simulink model "DcMotorSimulink"  (R2025a)
settings: Solver=FixedStepAuto  StartTime=0.0  StopTime=10  FixedStep=1e-4  RelTol=1e-3
undefined symbols (not defined in the file): bm, Jm, Kphi, La, Ra
settings Model: DataDictionary=DcMotor.sldd  Creator=tecnicomcbti  LastModifiedBy=tecnicomcbti
settings SolverCC: ConcurrentTasks=on  PositivePriorityOrder=on
settings OptimizationCC: BlockReduction=off  OptimizeBlockIOStorage=off
settings DebuggingCC: AlgebraicLoopMsg=none  TasksWithSamePriorityMsg=none
settings HardwareCC: ProdBitPerLong=64.0  ProdLongLongMode=on  ProdHWDeviceType=Intel->x86-64 (Linux 64)
settings RTWCC: SystemTargetFile=speedgoat.tlc  TemplateMakefile=slrealtime_default_tmf  Toolchain=Simulink Real-Time Toolchain  BuildConfiguration=Faster Runs  CodeExecutionProfiling=on  TargetLang=C++  Description=Speedgoat Real-Time Target Machine
settings SimulinkRealTimeTargetCC: SLRTFileLogMaxRuns=1.0  ExtModeMaxTrigDuration=10.0  ExtModeStaticAllocSize=1000000.0  ExtModeTransport=0.0  MultiwordLength=2048.0  DynamicStringBufferSize=256.0  PreserveMATLABNamespacesInGeneratedCode=on  SubcomponentCodeInterfacePackaging=Reusable function  InstructionSetFMA=off  LogToMDFFile=off

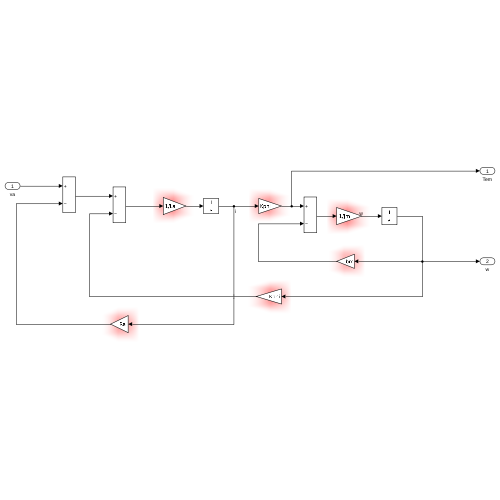
[thumbnail: Simulink's stored preview of the top-level diagram]
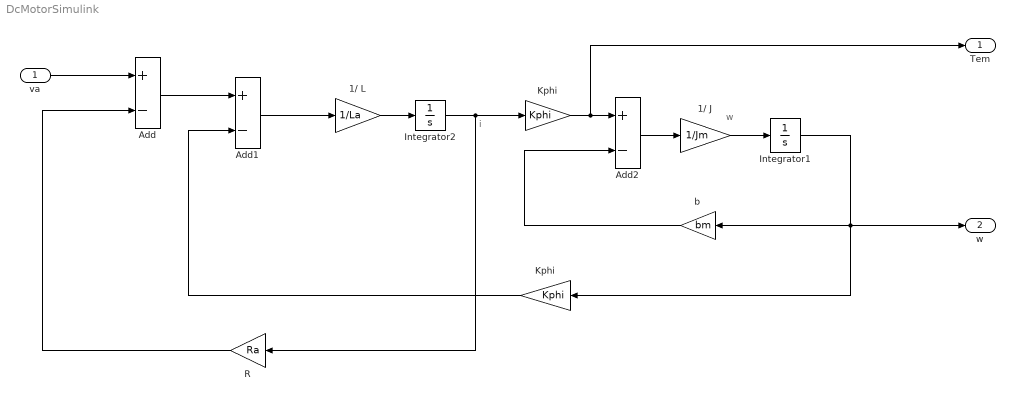
== system DcMotorSimulink ==
  note: w
  note: i
  va : Inport
  1/ J : Gain  Gain=1/Jm
  1/ L : Gain  Gain=1/La
  Add : Sum  Inputs=+-
  Add1 : Sum  Inputs=+-
  Add2 : Sum  Inputs=+-
  Integrator1 : Integrator
  Integrator2 : Integrator
  Kphi : Gain  Gain=Kphi
  "Kphi " : Gain  Gain=Kphi
  R : Gain  Gain=Ra
  b : Gain  Gain=bm
  Tem : Outport
  w : Outport  Port=2
  wires:
  b/1 -> Add2/2
  1/ L/1 -> Integrator2/1
  1/ J/1 -> Integrator1/1
  Integrator2/1 -> R/1, Kphi/1
  Add1/1 -> 1/ L/1
  Kphi/1 -> Tem/1, Add2/1
  Integrator1/1 -> w/1, "Kphi "/1, b/1
  Add2/1 -> 1/ J/1
  R/1 -> Add/2
  Add/1 -> Add1/1
  "Kphi "/1 -> Add1/2
  va/1 -> Add/1
